simulink model "gm_CIC_decimator_HDL_model"  (R2018b)
settings: Solver=FixedStepAuto  StartTime=0.0  StopTime=10  RelTol=1e-3  EnableMultiTasking=on
undefined symbols (not defined in the file or in its folder): DiscIntNeverNeededParam, Fs, ftest1, ftest2, ftest3, R
libraries: hdlsllib x4, dspsrcs4 x3, simulink x2, commchan3 x1
settings Model: Creator=MrGoshak  LastModifiedBy=MrGoshak
settings OptimizationCC: BlockReduction=off  ConditionallyExecuteInputs=off
settings DebuggingCC: InheritedTsInSrcMsg=none
settings HardwareCC: ProdBitPerPointer=32  ProdBitPerSizeT=32  ProdBitPerPtrDiffT=32  ProdLargestAtomicFloat=None  ProdIntDivRoundTo=Undefined  ProdEndianess=Unspecified  ProdWordSize=32  ProdHWDeviceType=ASIC/FPGA->ASIC/FPGA  TargetBitPerPointer=64  TargetBitPerSizeT=64  TargetBitPerPtrDiffT=64  TargetLongLongMode=on  TargetIntDivRoundTo=Zero  TargetEndianess=LittleEndian  TargetWordSize=64  TargetHWDeviceType=Custom Processor->MATLAB Host Computer  ProdEqTarget=off

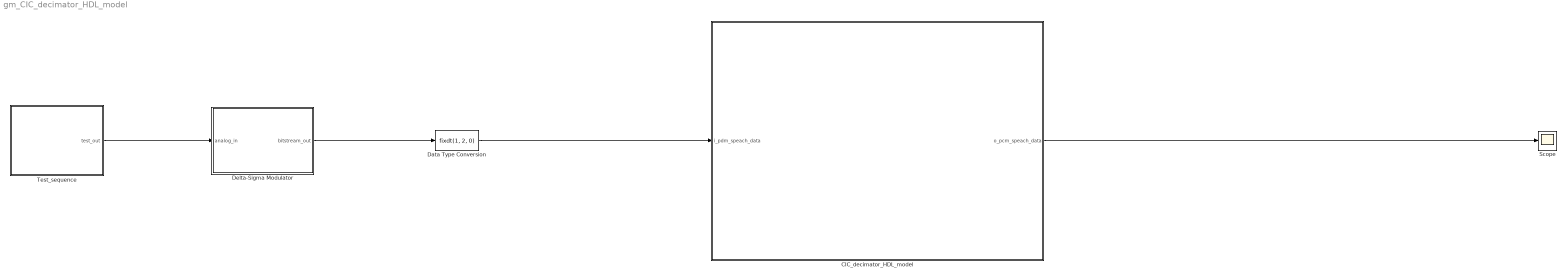
== system gm_CIC_decimator_HDL_model ==
  CIC_decimator_HDL_model : Subsystem
  Data Type Conversion : DataTypeConversion  OutDataTypeStr=fixdt(1, 2, 0)
  "Delta-Sigma Modulator " : Subsystem
  Scope : Scope
  "Test_sequence " : Subsystem
  wires:
  CIC_decimator_HDL_model/1(o_pcm_speach_data) -> Scope/1
  Data Type Conversion/1 -> CIC_decimator_HDL_model/1(i_pdm_speach_data)
  "Delta-Sigma Modulator "/1(bitstream_out) -> Data Type Conversion/1
  "Test_sequence "/1(test_out) -> "Delta-Sigma Modulator "/1(analog_in)

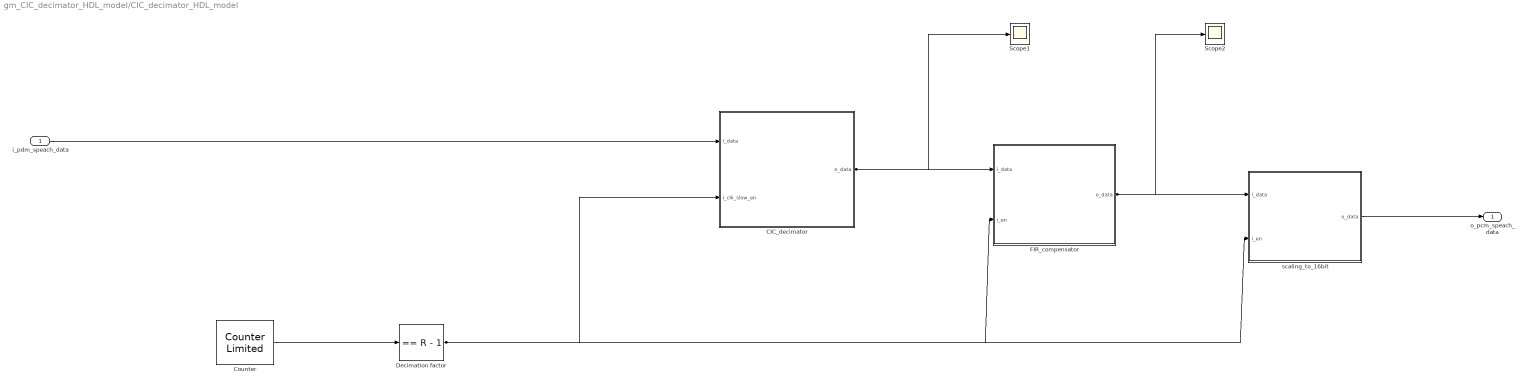
== system gm_CIC_decimator_HDL_model/CIC_decimator_HDL_model ==
  i_pdm_speach_data : Inport  OutDataTypeStr=fixdt(1, 2, 0)  PortDimensions=1  SampleTime=5e-07
  CIC_decimator : Subsystem
  "Counter " : simulink/Sources/Counter Limited  uplimit=R - 1  tsamp=1/Fs
  Decimation factor : simulink/Logic and Bit Operations/Compare To Constant  relop===  const=R - 1  OutDataTypeStr=boolean
  FIR_compensator : Subsystem
  Scope1 : Scope
  Scope2 : Scope
  scaling_to_16bit : Subsystem
  o_pcm_speach_data : Outport
  wires:
  i_pdm_speach_data/1 -> CIC_decimator/1(i_data)
  CIC_decimator/1(o_data) -> Scope1/1, FIR_compensator/1(i_data)
  "Counter "/1 -> Decimation factor/1
  Decimation factor/1 -> CIC_decimator/2(i_clk_slow_en), FIR_compensator/2(i_en), scaling_to_16bit/2(i_en)
  FIR_compensator/1(o_data) -> Scope2/1, scaling_to_16bit/1(i_data)
  scaling_to_16bit/1(o_data) -> o_pcm_speach_data/1

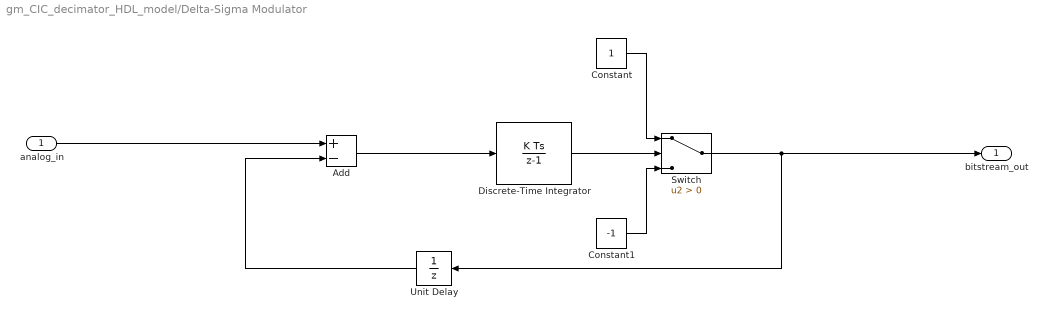
== system gm_CIC_decimator_HDL_model/Delta-Sigma Modulator  ==
  analog_in : Inport
  Add : Sum  Inputs=+-
  Constant : Constant
  Constant1 : Constant  Value=-1
  Discrete-Time Integrator : DiscreteIntegrator  SampleTime=-1  ICPrevOutput=DiscIntNeverNeededParam  ICPrevScaledInput=DiscIntNeverNeededParam
  Switch : Switch  Criteria=u2 > Threshold
  Unit Delay : UnitDelay  SampleTime=-1
  bitstream_out : Outport
  wires:
  Switch/1 -> Unit Delay/1, bitstream_out/1
  Constant/1 -> Switch/1
  Constant1/1 -> Switch/3
  Add/1 -> Discrete-Time Integrator/1
  analog_in/1 -> Add/1
  Discrete-Time Integrator/1 -> Switch/2
  Unit Delay/1 -> Add/2

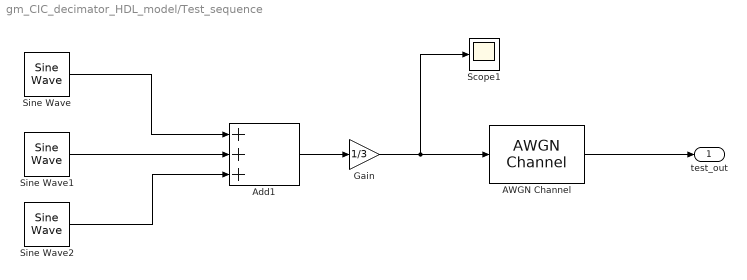
== system gm_CIC_decimator_HDL_model/Test_sequence  ==
  AWGN Channel : commchan3/AWGN Channel  InputProcessing=Columns as channels (frame based)  seed=67  noiseMode="Signal to noise ratio  (SNR)"  EbNodB=10  EsNodB=10  SNRdB=40  bitsPerSym=1  Ps=1  Tsym=1  variance=1
  Add1 : Sum  Inputs=+++
  Gain : Gain  Gain=1/3
  Scope1 : Scope
  Sine Wave : dspsrcs4/Sine Wave  Amplitude=1  Frequency=ftest1  Phase=0  SampleMode=Discrete  OutComplex=Real  CompMethod=Trigonometric fcn  TableSize=Speed  SampleTime=1/Fs  SamplesPerFrame=1  ResetState=Restart at time zero  OutputFrames=off  dataType=double  wordLen=16  udDataType=sfix(16)  fracBitsMode=User-defined  numFracBits=0  OutDataTypeStr=double  LastOutDataTypeStr=double
  Sine Wave1 : dspsrcs4/Sine Wave  Amplitude=1  Frequency=ftest2  Phase=0  SampleMode=Discrete  OutComplex=Real  CompMethod=Trigonometric fcn  TableSize=Speed  SampleTime=1/Fs  SamplesPerFrame=1  ResetState=Restart at time zero  OutputFrames=off  dataType=double  wordLen=16  udDataType=sfix(16)  fracBitsMode=Best precision  numFracBits=15  OutDataTypeStr=double  LastOutDataTypeStr=double
  Sine Wave2 : dspsrcs4/Sine Wave  Amplitude=1  Frequency=ftest3  Phase=0  SampleMode=Discrete  OutComplex=Real  CompMethod=Trigonometric fcn  TableSize=Speed  SampleTime=1/Fs  SamplesPerFrame=1  ResetState=Restart at time zero  OutputFrames=off  dataType=double  wordLen=16  udDataType=sfix(16)  fracBitsMode=Best precision  numFracBits=15  OutDataTypeStr=double  LastOutDataTypeStr=double
  test_out : Outport
  wires:
  AWGN Channel/1 -> test_out/1
  Sine Wave1/1 -> Add1/2
  Gain/1 -> Scope1/1, AWGN Channel/1
  Add1/1 -> Gain/1
  Sine Wave/1 -> Add1/1
  Sine Wave2/1 -> Add1/3

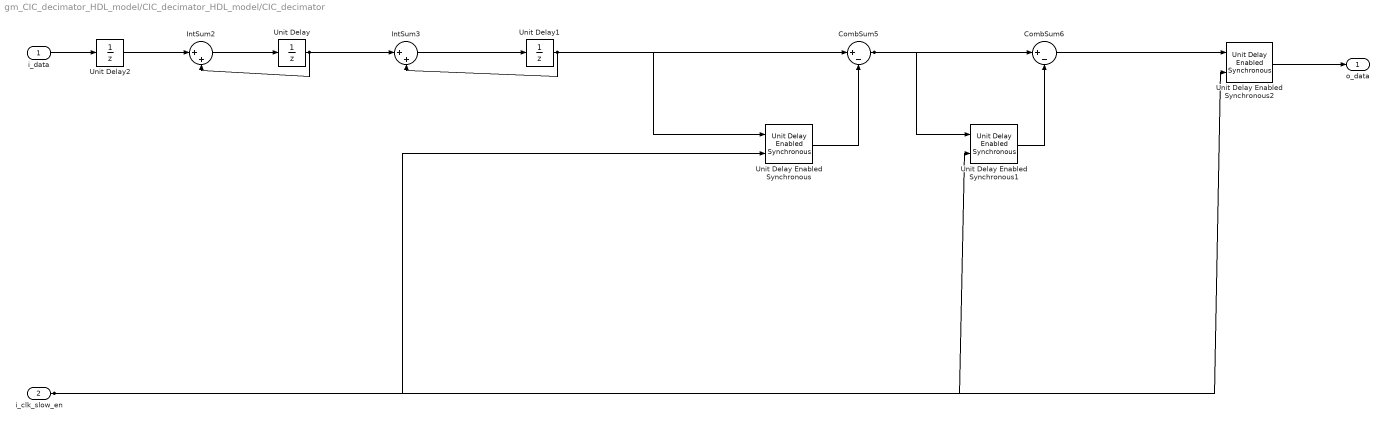
== system gm_CIC_decimator_HDL_model/CIC_decimator_HDL_model/CIC_decimator ==
  i_data : Inport  OutDataTypeStr=fixdt(1, 2, 0)  PortDimensions=1  SampleTime=5e-07
  i_clk_slow_en : Inport  Port=2  OutDataTypeStr=boolean  PortDimensions=1  SampleTime=5e-07
  CombSum5 : Sum  Inputs=|+-  OutDataTypeStr=CIC_data_type
  CombSum6 : Sum  Inputs=|+-  OutDataTypeStr=CIC_data_type
  IntSum2 : Sum  Inputs=|++  OutDataTypeStr=CIC_data_type
  IntSum3 : Sum  Inputs=|++  OutDataTypeStr=CIC_data_type
  Unit Delay : UnitDelay  SampleTime=-1
  Unit Delay Enabled Synchronous : hdlsllib/Discrete/Unit Delay Enabled Synchronous  InitialCondition=0.0  SampleTime=-1
      settings: SourceProductName=HDL Coder  SourceProductBaseCode=HD
  Unit Delay Enabled Synchronous1 : hdlsllib/Discrete/Unit Delay Enabled Synchronous  InitialCondition=0.0  SampleTime=-1
      settings: SourceProductName=HDL Coder  SourceProductBaseCode=HD
  Unit Delay Enabled Synchronous2 : hdlsllib/Discrete/Unit Delay Enabled Synchronous  InitialCondition=0.0  SampleTime=-1
      settings: SourceProductName=HDL Coder  SourceProductBaseCode=HD
  Unit Delay1 : UnitDelay  SampleTime=-1
  Unit Delay2 : UnitDelay  SampleTime=-1
  o_data : Outport
  wires:
  CombSum5/1 -> CombSum6/1, Unit Delay Enabled Synchronous1/1
  CombSum6/1 -> Unit Delay Enabled Synchronous2/1
  Unit Delay/1 -> IntSum2/2, IntSum3/1
  Unit Delay Enabled Synchronous/1 -> CombSum5/2
  Unit Delay Enabled Synchronous1/1 -> CombSum6/2
  Unit Delay Enabled Synchronous2/1 -> o_data/1
  Unit Delay1/1 -> CombSum5/1, Unit Delay Enabled Synchronous/1, IntSum3/2
  Unit Delay2/1 -> IntSum2/1
  i_data/1 -> Unit Delay2/1
  i_clk_slow_en/1 -> Unit Delay Enabled Synchronous2/2, Unit Delay Enabled Synchronous1/2, Unit Delay Enabled Synchronous/2
  IntSum2/1 -> Unit Delay/1
  IntSum3/1 -> Unit Delay1/1

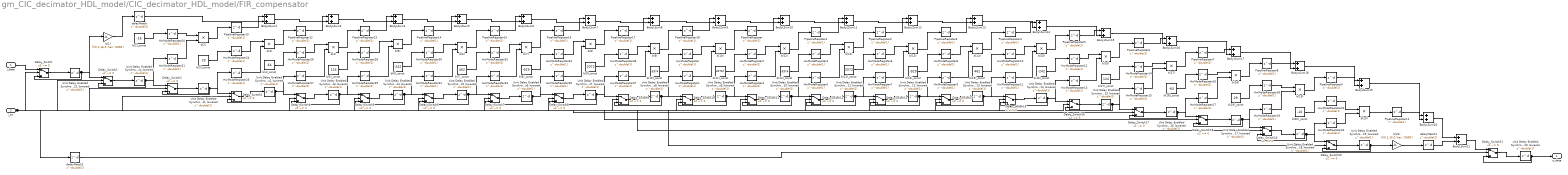
== system gm_CIC_decimator_HDL_model/CIC_decimator_HDL_model/FIR_compensator ==
  i_data : Inport  OutDataTypeStr=fixdt(1, 15, 0)  PortDimensions=1  SampleTime=5e-07
  i_en : Inport  Port=2  OutDataTypeStr=boolean  PortDimensions=1  SampleTime=5e-07
  BodyLSum{2..21} (20 alike) : Sum  AccumDataTypeStr=fixdt(1, 31, 0)  OutDataTypeStr=fixdt(1, 31, 0)  SampleTime=5e-07  SaturateOnIntegerOverflow=on
  Delay_Switch{,1..20} (21 alike) : Switch  Criteria=u2 ~= 0  Threshold=double(0)  OutDataTypeStr=fixdt(1, 15, 0)  SampleTime=5e-07
  Delay_Switch21 : Switch  Criteria=u2 ~= 0  Threshold=double(0)  OutDataTypeStr=fixdt(1, 31, 0)  SampleTime=5e-07
  HwModeRegister{,1..37} (38 alike) : Delay  DelayLength=double(1)  InitialCondition=0  InputProcessing=Inherited  SampleTime=5e-07
  PipelineRegister{,1..18} (19 alike) : Delay  DelayLength=double(1)  InitialCondition=0  InputProcessing=Inherited  SampleTime=5e-07
  Unit Delay Enabled Synchronous10_lowered : Delay  DelayLength=double(1)  InitialCondition=0  InputProcessing=Inherited  SampleTime=5e-07
  Unit Delay Enabled Synchronous11_lowered : Delay  DelayLength=double(1)  InitialCondition=0  InputProcessing=Inherited  SampleTime=5e-07
  Unit Delay Enabled Synchronous12_lowered : Delay  DelayLength=double(1)  InitialCondition=0  InputProcessing=Inherited  SampleTime=5e-07
  Unit Delay Enabled Synchronous13_lowered : Delay  DelayLength=double(1)  InitialCondition=0  InputProcessing=Inherited  SampleTime=5e-07
  Unit Delay Enabled Synchronous14_lowered : Delay  DelayLength=double(1)  InitialCondition=0  InputProcessing=Inherited  SampleTime=5e-07
  Unit Delay Enabled Synchronous15_lowered : Delay  DelayLength=double(1)  InitialCondition=0  InputProcessing=Inherited  SampleTime=5e-07
  Unit Delay Enabled Synchronous16_lowered : Delay  DelayLength=double(1)  InitialCondition=0  InputProcessing=Inherited  SampleTime=5e-07
  Unit Delay Enabled Synchronous17_lowered : Delay  DelayLength=double(1)  InitialCondition=0  InputProcessing=Inherited  SampleTime=5e-07
  Unit Delay Enabled Synchronous18_lowered : Delay  DelayLength=double(1)  InitialCondition=0  InputProcessing=Inherited  SampleTime=5e-07
  Unit Delay Enabled Synchronous19_lowered : Delay  DelayLength=double(1)  InitialCondition=0  InputProcessing=Inherited  SampleTime=5e-07
  Unit Delay Enabled Synchronous1_lowered : Delay  DelayLength=double(1)  InitialCondition=0  InputProcessing=Inherited  SampleTime=5e-07
  Unit Delay Enabled Synchronous20_lowered : Delay  DelayLength=double(1)  InitialCondition=0  InputProcessing=Inherited  SampleTime=5e-07
  Unit Delay Enabled Synchronous21_lowered : Delay  DelayLength=double(1)  InitialCondition=0  InputProcessing=Inherited  SampleTime=5e-07
  Unit Delay Enabled Synchronous2_lowered : Delay  DelayLength=double(1)  InitialCondition=0  InputProcessing=Inherited  SampleTime=5e-07
  Unit Delay Enabled Synchronous3_lowered : Delay  DelayLength=double(1)  InitialCondition=0  InputProcessing=Inherited  SampleTime=5e-07
  Unit Delay Enabled Synchronous4_lowered : Delay  DelayLength=double(1)  InitialCondition=0  InputProcessing=Inherited  SampleTime=5e-07
  Unit Delay Enabled Synchronous5_lowered : Delay  DelayLength=double(1)  InitialCondition=0  InputProcessing=Inherited  SampleTime=5e-07
  Unit Delay Enabled Synchronous6_lowered : Delay  DelayLength=double(1)  InitialCondition=0  InputProcessing=Inherited  SampleTime=5e-07
  Unit Delay Enabled Synchronous7_lowered : Delay  DelayLength=double(1)  InitialCondition=0  InputProcessing=Inherited  SampleTime=5e-07
  Unit Delay Enabled Synchronous8_lowered : Delay  DelayLength=double(1)  InitialCondition=0  InputProcessing=Inherited  SampleTime=5e-07
  Unit Delay Enabled Synchronous9_lowered : Delay  DelayLength=double(1)  InitialCondition=0  InputProcessing=Inherited  SampleTime=5e-07
  Unit Delay Enabled Synchronous_lowered : Delay  DelayLength=double(1)  InitialCondition=0  InputProcessing=Inherited  SampleTime=5e-07
  b(1) : Gain  Gain=fi(0,1,16,0,'hex','0008')  ParamDataTypeStr=fixdt(1, 16, 0)  OutDataTypeStr=fixdt(1, 31, 0)  SampleTime=5e-07  SaturateOnIntegerOverflow=on
  b(10) : Product  Inputs=**  OutDataTypeStr=fixdt(1, 31, 0)  SampleTime=5e-07  SaturateOnIntegerOverflow=on
  b(10)_const : Constant  Value=-5974  OutDataTypeStr=int16  SampleTime=-1
  b(11) : Product  Inputs=**  OutDataTypeStr=fixdt(1, 31, 0)  SampleTime=5e-07  SaturateOnIntegerOverflow=on
  b(11)_const : Constant  Value=32767  OutDataTypeStr=int16  SampleTime=-1
  b(12) : Product  Inputs=**  OutDataTypeStr=fixdt(1, 31, 0)  SampleTime=5e-07  SaturateOnIntegerOverflow=on
  b(12)_const : Constant  Value=-5974  OutDataTypeStr=int16  SampleTime=-1
  b(13) : Product  Inputs=**  OutDataTypeStr=fixdt(1, 31, 0)  SampleTime=5e-07  SaturateOnIntegerOverflow=on
  b(13)_const : Constant  Value=2072  OutDataTypeStr=int16  SampleTime=-1
  b(14) : Product  Inputs=**  OutDataTypeStr=fixdt(1, 31, 0)  SampleTime=5e-07  SaturateOnIntegerOverflow=on
  b(14)_const : Constant  Value=-929  OutDataTypeStr=int16  SampleTime=-1
  b(15) : Product  Inputs=**  OutDataTypeStr=fixdt(1, 31, 0)  SampleTime=5e-07  SaturateOnIntegerOverflow=on
  b(15)_const : Constant  Value=462  OutDataTypeStr=int16  SampleTime=-1
  b(16) : Product  Inputs=**  OutDataTypeStr=fixdt(1, 31, 0)  SampleTime=5e-07  SaturateOnIntegerOverflow=on
  b(16)_const : Constant  Value=-242  OutDataTypeStr=int16  SampleTime=-1
  b(17) : Product  Inputs=**  OutDataTypeStr=fixdt(1, 31, 0)  SampleTime=5e-07  SaturateOnIntegerOverflow=on
  b(17)_const : Constant  Value=124  OutDataTypeStr=int16  SampleTime=-1
  b(18) : Product  Inputs=**  OutDataTypeStr=fixdt(1, 31, 0)  SampleTime=5e-07  SaturateOnIntegerOverflow=on
  b(18)_const : Constant  Value=-64  OutDataTypeStr=int16  SampleTime=-1
  b(19) : Product  Inputs=**  OutDataTypeStr=fixdt(1, 31, 0)  SampleTime=5e-07  SaturateOnIntegerOverflow=on
  b(19)_const : Constant  Value=29  OutDataTypeStr=int16  SampleTime=-1
  b(2) : Product  Inputs=**  OutDataTypeStr=fixdt(1, 31, 0)  SampleTime=5e-07  SaturateOnIntegerOverflow=on
  b(2)_const : Constant  Value=-16  OutDataTypeStr=int16  SampleTime=-1
  b(20) : Product  Inputs=**  OutDataTypeStr=fixdt(1, 31, 0)  SampleTime=5e-07  SaturateOnIntegerOverflow=on
  b(20)_const : Constant  Value=-16  OutDataTypeStr=int16  SampleTime=-1
  b(21) : Gain  Gain=fi(0,1,16,0,'hex','0008')  ParamDataTypeStr=fixdt(1, 16, 0)  OutDataTypeStr=fixdt(1, 31, 0)  SampleTime=5e-07  SaturateOnIntegerOverflow=on
  b(3) : Product  Inputs=**  OutDataTypeStr=fixdt(1, 31, 0)  SampleTime=5e-07  SaturateOnIntegerOverflow=on
  b(3)_const : Constant  Value=29  OutDataTypeStr=int16  SampleTime=-1
  b(4) : Product  Inputs=**  OutDataTypeStr=fixdt(1, 31, 0)  SampleTime=5e-07  SaturateOnIntegerOverflow=on
  b(4)_const : Constant  Value=-64  OutDataTypeStr=int16  SampleTime=-1
  b(5) : Product  Inputs=**  OutDataTypeStr=fixdt(1, 31, 0)  SampleTime=5e-07  SaturateOnIntegerOverflow=on
  b(5)_const : Constant  Value=124  OutDataTypeStr=int16  SampleTime=-1
  b(6) : Product  Inputs=**  OutDataTypeStr=fixdt(1, 31, 0)  SampleTime=5e-07  SaturateOnIntegerOverflow=on
  b(6)_const : Constant  Value=-242  OutDataTypeStr=int16  SampleTime=-1
  b(7) : Product  Inputs=**  OutDataTypeStr=fixdt(1, 31, 0)  SampleTime=5e-07  SaturateOnIntegerOverflow=on
  b(7)_const : Constant  Value=462  OutDataTypeStr=int16  SampleTime=-1
  b(8) : Product  Inputs=**  OutDataTypeStr=fixdt(1, 31, 0)  SampleTime=5e-07  SaturateOnIntegerOverflow=on
  b(8)_const : Constant  Value=-929  OutDataTypeStr=int16  SampleTime=-1
  b(9) : Product  Inputs=**  OutDataTypeStr=fixdt(1, 31, 0)  SampleTime=5e-07  SaturateOnIntegerOverflow=on
  b(9)_const : Constant  Value=2072  OutDataTypeStr=int16  SampleTime=-1
  delayMatch : Delay  DelayLength=double(2)  InitialCondition=0  InputProcessing=Inherited  SampleTime=5e-07
  delayMatch1 : Delay  DelayLength=double(2)  InitialCondition=0  InputProcessing=Inherited  SampleTime=5e-07
  delayMatch2 : Delay  DelayLength=double(2)  InitialCondition=0  InputProcessing=Inherited  SampleTime=5e-07
  o_data : Outport
  wires:
  delayMatch2/1 -> Delay_Switch21/2
  BodyLSum10/1 -> BodyLSum11/2
  BodyLSum11/1 -> BodyLSum12/2
  BodyLSum12/1 -> BodyLSum13/2
  BodyLSum13/1 -> BodyLSum14/2
  BodyLSum14/1 -> BodyLSum15/2
  BodyLSum15/1 -> BodyLSum16/2
  BodyLSum16/1 -> BodyLSum17/2
  BodyLSum17/1 -> BodyLSum18/2
  BodyLSum18/1 -> BodyLSum19/2
  BodyLSum19/1 -> BodyLSum20/2
  BodyLSum2/1 -> BodyLSum3/2
  BodyLSum20/1 -> BodyLSum21/1
  BodyLSum21/1 -> Delay_Switch21/1
  BodyLSum3/1 -> BodyLSum4/2
  BodyLSum4/1 -> BodyLSum5/2
  BodyLSum5/1 -> BodyLSum6/2
  BodyLSum6/1 -> BodyLSum7/2
  BodyLSum7/1 -> BodyLSum8/2
  BodyLSum8/1 -> BodyLSum9/2
  BodyLSum9/1 -> BodyLSum10/2
  Unit Delay Enabled Synchronous_lowered/1 -> Delay_Switch1/3, Delay_Switch2/1, HwModeRegister21/1
  Unit Delay Enabled Synchronous1_lowered/1 -> Delay_Switch2/3, Delay_Switch3/1, HwModeRegister25/1
  Unit Delay Enabled Synchronous10_lowered/1 -> Delay_Switch11/3, Delay_Switch12/1, HwModeRegister5/1
  Unit Delay Enabled Synchronous11_lowered/1 -> Delay_Switch12/3, Delay_Switch13/1, HwModeRegister7/1
  Unit Delay Enabled Synchronous12_lowered/1 -> Delay_Switch13/3, Delay_Switch14/1, HwModeRegister9/1
  Unit Delay Enabled Synchronous13_lowered/1 -> Delay_Switch14/3, Delay_Switch15/1, HwModeRegister11/1
  Unit Delay Enabled Synchronous14_lowered/1 -> Delay_Switch15/3, Delay_Switch16/1, HwModeRegister13/1
  Unit Delay Enabled Synchronous15_lowered/1 -> Delay_Switch16/3, Delay_Switch17/1, HwModeRegister15/1
  Unit Delay Enabled Synchronous16_lowered/1 -> Delay_Switch17/3, Delay_Switch18/1, HwModeRegister17/1
  Unit Delay Enabled Synchronous17_lowered/1 -> Delay_Switch18/3, Delay_Switch19/1, HwModeRegister19/1
  Unit Delay Enabled Synchronous18_lowered/1 -> Delay_Switch19/3, Delay_Switch20/1, HwModeRegister23/1
  Unit Delay Enabled Synchronous19_lowered/1 -> b(21)/1, Delay_Switch20/3
  Unit Delay Enabled Synchronous2_lowered/1 -> Delay_Switch3/3, Delay_Switch4/1, HwModeRegister27/1
  Unit Delay Enabled Synchronous21_lowered/1 -> b(1)/1, Delay_Switch/3, Delay_Switch1/1
  Unit Delay Enabled Synchronous3_lowered/1 -> Delay_Switch4/3, Delay_Switch5/1, HwModeRegister29/1
  Unit Delay Enabled Synchronous4_lowered/1 -> Delay_Switch5/3, Delay_Switch6/1, HwModeRegister31/1
  Unit Delay Enabled Synchronous5_lowered/1 -> Delay_Switch6/3, Delay_Switch7/1, HwModeRegister33/1
  Unit Delay Enabled Synchronous6_lowered/1 -> Delay_Switch7/3, Delay_Switch8/1, HwModeRegister35/1
  Unit Delay Enabled Synchronous7_lowered/1 -> Delay_Switch8/3, Delay_Switch9/1, HwModeRegister37/1
  Unit Delay Enabled Synchronous8_lowered/1 -> Delay_Switch9/3, Delay_Switch10/1, HwModeRegister1/1
  Unit Delay Enabled Synchronous9_lowered/1 -> Delay_Switch10/3, Delay_Switch11/1, HwModeRegister3/1
  delayMatch/1 -> BodyLSum2/2
  PipelineRegister/1 -> BodyLSum10/1
  PipelineRegister1/1 -> BodyLSum11/1
  PipelineRegister2/1 -> BodyLSum12/1
  PipelineRegister3/1 -> BodyLSum13/1
  PipelineRegister4/1 -> BodyLSum14/1
  PipelineRegister5/1 -> BodyLSum15/1
  PipelineRegister6/1 -> BodyLSum16/1
  PipelineRegister7/1 -> BodyLSum17/1
  PipelineRegister8/1 -> BodyLSum18/1
  PipelineRegister9/1 -> BodyLSum19/1
  PipelineRegister10/1 -> BodyLSum2/1
  PipelineRegister11/1 -> BodyLSum20/1
  delayMatch1/1 -> BodyLSum21/2
  PipelineRegister12/1 -> BodyLSum3/1
  PipelineRegister13/1 -> BodyLSum4/1
  PipelineRegister14/1 -> BodyLSum5/1
  PipelineRegister15/1 -> BodyLSum6/1
  PipelineRegister16/1 -> BodyLSum7/1
  PipelineRegister17/1 -> BodyLSum8/1
  PipelineRegister18/1 -> BodyLSum9/1
  b(10)_const/1 -> HwModeRegister/1
  b(11)_const/1 -> HwModeRegister2/1
  b(12)_const/1 -> HwModeRegister4/1
  b(13)_const/1 -> HwModeRegister6/1
  b(14)_const/1 -> HwModeRegister8/1
  b(15)_const/1 -> HwModeRegister10/1
  b(16)_const/1 -> HwModeRegister12/1
  b(17)_const/1 -> HwModeRegister14/1
  b(18)_const/1 -> HwModeRegister16/1
  b(19)_const/1 -> HwModeRegister18/1
  b(2)_const/1 -> HwModeRegister20/1
  b(20)_const/1 -> HwModeRegister22/1
  b(3)_const/1 -> HwModeRegister24/1
  b(4)_const/1 -> HwModeRegister26/1
  b(5)_const/1 -> HwModeRegister28/1
  b(6)_const/1 -> HwModeRegister30/1
  b(7)_const/1 -> HwModeRegister32/1
  b(8)_const/1 -> HwModeRegister34/1
  b(9)_const/1 -> HwModeRegister36/1
  i_data/1 -> Delay_Switch/1
  i_en/1 -> delayMatch2/1, Delay_Switch/2, Delay_Switch1/2, Delay_Switch2/2, Delay_Switch3/2, Delay_Switch4/2, Delay_Switch5/2, Delay_Switch6/2, Delay_Switch7/2, Delay_Switch8/2, Delay_Switch9/2, Delay_Switch10/2, Delay_Switch11/2, Delay_Switch12/2, Delay_Switch13/2, Delay_Switch14/2, Delay_Switch15/2, Delay_Switch16/2, Delay_Switch17/2, Delay_Switch18/2, Delay_Switch19/2, Delay_Switch20/2
  b(1)/1 -> delayMatch/1
  b(21)/1 -> delayMatch1/1
  Delay_Switch/1 -> Unit Delay Enabled Synchronous21_lowered/1
  Delay_Switch1/1 -> Unit Delay Enabled Synchronous_lowered/1
  Delay_Switch2/1 -> Unit Delay Enabled Synchronous1_lowered/1
  Delay_Switch3/1 -> Unit Delay Enabled Synchronous2_lowered/1
  Delay_Switch4/1 -> Unit Delay Enabled Synchronous3_lowered/1
  Delay_Switch5/1 -> Unit Delay Enabled Synchronous4_lowered/1
  Delay_Switch6/1 -> Unit Delay Enabled Synchronous5_lowered/1
  Delay_Switch7/1 -> Unit Delay Enabled Synchronous6_lowered/1
  Delay_Switch8/1 -> Unit Delay Enabled Synchronous7_lowered/1
  Delay_Switch9/1 -> Unit Delay Enabled Synchronous8_lowered/1
  Delay_Switch10/1 -> Unit Delay Enabled Synchronous9_lowered/1
  Delay_Switch11/1 -> Unit Delay Enabled Synchronous10_lowered/1
  Delay_Switch12/1 -> Unit Delay Enabled Synchronous11_lowered/1
  Delay_Switch13/1 -> Unit Delay Enabled Synchronous12_lowered/1
  Delay_Switch14/1 -> Unit Delay Enabled Synchronous13_lowered/1
  Delay_Switch15/1 -> Unit Delay Enabled Synchronous14_lowered/1
  Delay_Switch16/1 -> Unit Delay Enabled Synchronous15_lowered/1
  Delay_Switch17/1 -> Unit Delay Enabled Synchronous16_lowered/1
  Delay_Switch18/1 -> Unit Delay Enabled Synchronous17_lowered/1
  Delay_Switch19/1 -> Unit Delay Enabled Synchronous18_lowered/1
  Delay_Switch20/1 -> Unit Delay Enabled Synchronous19_lowered/1
  Delay_Switch21/1 -> Unit Delay Enabled Synchronous20_lowered/1
  Unit Delay Enabled Synchronous20_lowered/1 -> Delay_Switch21/3, o_data/1
  b(10)/1 -> PipelineRegister/1
  HwModeRegister/1 -> b(10)/1
  HwModeRegister1/1 -> b(10)/2
  b(11)/1 -> PipelineRegister1/1
  HwModeRegister2/1 -> b(11)/1
  HwModeRegister3/1 -> b(11)/2
  b(12)/1 -> PipelineRegister2/1
  HwModeRegister4/1 -> b(12)/1
  HwModeRegister5/1 -> b(12)/2
  b(13)/1 -> PipelineRegister3/1
  HwModeRegister6/1 -> b(13)/1
  HwModeRegister7/1 -> b(13)/2
  b(14)/1 -> PipelineRegister4/1
  HwModeRegister8/1 -> b(14)/1
  HwModeRegister9/1 -> b(14)/2
  b(15)/1 -> PipelineRegister5/1
  HwModeRegister10/1 -> b(15)/1
  HwModeRegister11/1 -> b(15)/2
  b(16)/1 -> PipelineRegister6/1
  HwModeRegister12/1 -> b(16)/1
  HwModeRegister13/1 -> b(16)/2
  b(17)/1 -> PipelineRegister7/1
  HwModeRegister14/1 -> b(17)/1
  HwModeRegister15/1 -> b(17)/2
  b(18)/1 -> PipelineRegister8/1
  HwModeRegister16/1 -> b(18)/1
  HwModeRegister17/1 -> b(18)/2
  b(19)/1 -> PipelineRegister9/1
  HwModeRegister18/1 -> b(19)/1
  HwModeRegister19/1 -> b(19)/2
  b(2)/1 -> PipelineRegister10/1
  HwModeRegister20/1 -> b(2)/1
  HwModeRegister21/1 -> b(2)/2
  b(20)/1 -> PipelineRegister11/1
  HwModeRegister22/1 -> b(20)/1
  HwModeRegister23/1 -> b(20)/2
  b(3)/1 -> PipelineRegister12/1
  HwModeRegister24/1 -> b(3)/1
  HwModeRegister25/1 -> b(3)/2
  b(4)/1 -> PipelineRegister13/1
  HwModeRegister26/1 -> b(4)/1
  HwModeRegister27/1 -> b(4)/2
  b(5)/1 -> PipelineRegister14/1
  HwModeRegister28/1 -> b(5)/1
  HwModeRegister29/1 -> b(5)/2
  b(6)/1 -> PipelineRegister15/1
  HwModeRegister30/1 -> b(6)/1
  HwModeRegister31/1 -> b(6)/2
  b(7)/1 -> PipelineRegister16/1
  HwModeRegister32/1 -> b(7)/1
  HwModeRegister33/1 -> b(7)/2
  b(8)/1 -> PipelineRegister17/1
  HwModeRegister34/1 -> b(8)/1
  HwModeRegister35/1 -> b(8)/2
  b(9)/1 -> PipelineRegister18/1
  HwModeRegister36/1 -> b(9)/1
  HwModeRegister37/1 -> b(9)/2

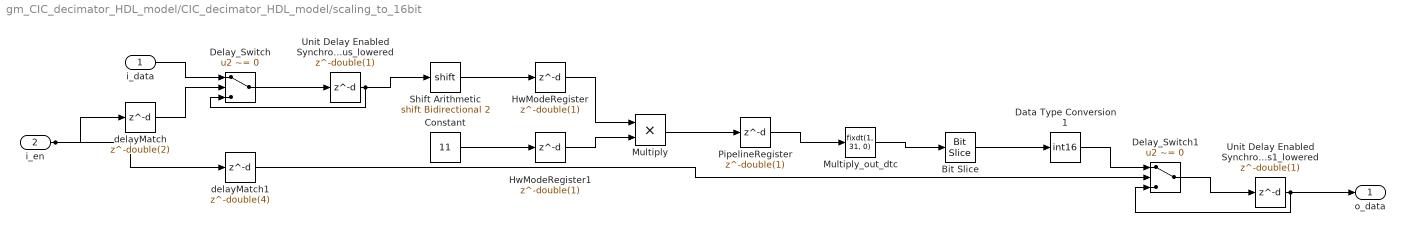
== system gm_CIC_decimator_HDL_model/CIC_decimator_HDL_model/scaling_to_16bit ==
  i_data : Inport  OutDataTypeStr=fixdt(1, 31, 0)  PortDimensions=1  SampleTime=5e-07
  i_en : Inport  Port=2  OutDataTypeStr=boolean  PortDimensions=1  SampleTime=5e-07
  Bit Slice : hdlsllib/Logic and Bit Operations/Bit Slice  lidx=double(30)  ridx=double(15)
  Constant : Constant  Value=11  OutDataTypeStr=uint8  SampleTime=-1
  Data Type Conversion1 : DataTypeConversion  OutDataTypeStr=int16  SampleTime=5e-07
  Delay_Switch : Switch  Criteria=u2 ~= 0  Threshold=double(0)  OutDataTypeStr=fixdt(1, 31, 0)  SampleTime=5e-07
  Delay_Switch1 : Switch  Criteria=u2 ~= 0  Threshold=double(0)  OutDataTypeStr=int16  SampleTime=5e-07
  HwModeRegister : Delay  DelayLength=double(1)  InitialCondition=0  InputProcessing=Inherited  SampleTime=5e-07
  HwModeRegister1 : Delay  DelayLength=double(1)  InitialCondition=0  InputProcessing=Inherited  SampleTime=5e-07
  Multiply : Product  Inputs=**  OutDataTypeStr=fixdt(1, 39, 0)  SampleTime=5e-07
  Multiply_out_dtc : DataTypeConversion  OutDataTypeStr=fixdt(1, 31, 0)  SampleTime=5e-07  SaturateOnIntegerOverflow=on
  PipelineRegister : Delay  DelayLength=double(1)  InitialCondition=0  InputProcessing=Inherited  SampleTime=5e-07
  Shift Arithmetic : ArithShift  BitShiftNumber=2  BinPtShiftNumber=double(0)
  Unit Delay Enabled Synchronous1_lowered : Delay  DelayLength=double(1)  InitialCondition=0  InputProcessing=Inherited  SampleTime=5e-07
  Unit Delay Enabled Synchronous_lowered : Delay  DelayLength=double(1)  InitialCondition=0  InputProcessing=Inherited  SampleTime=5e-07
  delayMatch : Delay  DelayLength=double(2)  InitialCondition=0  InputProcessing=Inherited  SampleTime=5e-07
  delayMatch1 : Delay  DelayLength=double(4)  InitialCondition=0  InputProcessing=Inherited  SampleTime=5e-07
  o_data : Outport
  wires:
  delayMatch/1 -> Delay_Switch/2
  Bit Slice/1 -> Data Type Conversion1/1
  Constant/1 -> HwModeRegister1/1
  Data Type Conversion1/1 -> Delay_Switch1/1
  Multiply_out_dtc/1 -> Bit Slice/1
  Shift Arithmetic/1 -> HwModeRegister/1
  PipelineRegister/1 -> Multiply_out_dtc/1
  i_data/1 -> Delay_Switch/1
  i_en/1 -> delayMatch1/1, delayMatch/1
  delayMatch1/1 -> Delay_Switch1/2
  Delay_Switch/1 -> Unit Delay Enabled Synchronous_lowered/1
  Unit Delay Enabled Synchronous_lowered/1 -> Delay_Switch/3, Shift Arithmetic/1
  Delay_Switch1/1 -> Unit Delay Enabled Synchronous1_lowered/1
  Unit Delay Enabled Synchronous1_lowered/1 -> Delay_Switch1/3, o_data/1
  Multiply/1 -> PipelineRegister/1
  HwModeRegister/1 -> Multiply/1
  HwModeRegister1/1 -> Multiply/2
